simulink model "test_control_lib_poly_ctr_w_aw"  (R2017a)
settings: Solver=VariableStepAuto  StartTime=0.0  StopTime=0.020*100  RelTol=1e-3
libraries: simulink x11
settings Model: Creator=CHIVFUR  LastModifiedBy=CHIVFUR

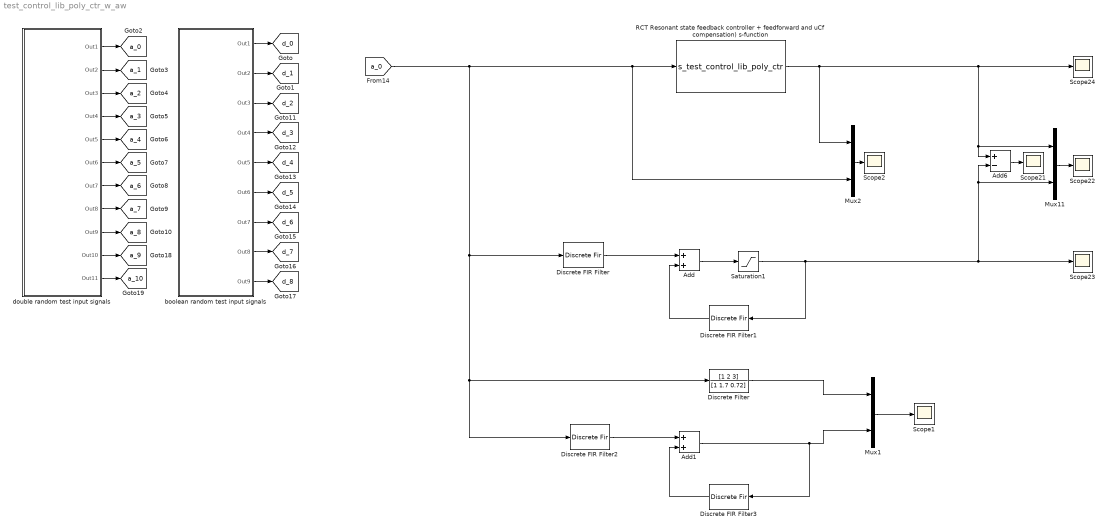
== system test_control_lib_poly_ctr_w_aw ==
  Add : Sum
  Add1 : Sum
  Add6 : Sum  Inputs=+-
  Discrete FIR Filter : DiscreteFir  Coefficients=[1 2 3]  SampleTime=1/30000
  Discrete FIR Filter1 : DiscreteFir  Coefficients=[0 -1.7 -0.72]  SampleTime=1/30000
  Discrete FIR Filter2 : DiscreteFir  Coefficients=[1 2 3]  SampleTime=1/30000
  Discrete FIR Filter3 : DiscreteFir  Coefficients=[0 -1.7 -0.72]  SampleTime=1/30000
  Discrete Filter : DiscreteFilter  Numerator=[1 2 3]  Denominator=[1 1.7 0.72]  SampleTime=1/30000
  Mux1 : Mux  Inputs=2
  Mux11 : Mux  Inputs=2
  Mux2 : Mux  Inputs=2
  RCT Resonant state feedback controller + feedforward and uCf compensation) s-function : S-Function  FunctionName=s_test_control_lib_poly_ctr  Parameters=1/30000,1.0  SFunctionDeploymentMode=off  EnableBusSupport=off
  Saturation1 : Saturate  UpperLimit=100  LowerLimit=-100
  Scope{1..2,21..24} (6 alike) : Scope
  boolean random test input signals : Subsystem
  double random test input signals : Subsystem
  tag scope: a_0=global, a_10=global, a_1=global, a_2=global, a_3=global, a_4=global, a_5=global, a_6=global, a_7=global, a_8=global, a_9=global, d_0=global, d_1=global, d_2=global, d_3=global, d_4=global, d_5=global, d_6=global, d_7=global, d_8=global
  wires:
  boolean random test input signals/2(Out2) -> [d_1]
  boolean random test input signals/1(Out1) -> [d_0]
  double random test input signals/1(Out1) -> [a_0]
  double random test input signals/2(Out2) -> [a_1]
  double random test input signals/3(Out3) -> [a_2]
  double random test input signals/4(Out4) -> [a_3]
  [a_0] -> Discrete FIR Filter/1, Discrete Filter/1, Discrete FIR Filter2/1, Mux2/2, RCT Resonant state feedback controller + feedforward and uCf compensation) s-function/1
  Add/1 -> Saturation1/1
  Add6/1 -> Scope21/1
  Mux11/1 -> Scope22/1
  double random test input signals/5(Out5) -> [a_4]
  double random test input signals/6(Out6) -> [a_5]
  double random test input signals/7(Out7) -> [a_6]
  double random test input signals/8(Out8) -> [a_7]
  double random test input signals/9(Out9) -> [a_8]
  boolean random test input signals/3(Out3) -> [d_2]
  boolean random test input signals/4(Out4) -> [d_3]
  boolean random test input signals/5(Out5) -> [d_4]
  boolean random test input signals/6(Out6) -> [d_5]
  boolean random test input signals/7(Out7) -> [d_6]
  boolean random test input signals/8(Out8) -> [d_7]
  boolean random test input signals/9(Out9) -> [d_8]
  double random test input signals/10(Out10) -> [a_9]
  double random test input signals/11(Out11) -> [a_10]
  Discrete FIR Filter1/1 -> Add/2
  RCT Resonant state feedback controller + feedforward and uCf compensation) s-function/1 -> Mux2/1, Scope24/1, Mux11/1, Add6/1
  Discrete FIR Filter/1 -> Add/1
  Discrete FIR Filter2/1 -> Add1/1
  Discrete FIR Filter3/1 -> Add1/2
  Discrete Filter/1 -> Mux1/1
  Add1/1 -> Discrete FIR Filter3/1, Mux1/2
  Mux1/1 -> Scope1/1
  Saturation1/1 -> Mux11/2, Add6/2, Scope23/1, Discrete FIR Filter1/1
  Mux2/1 -> Scope2/1

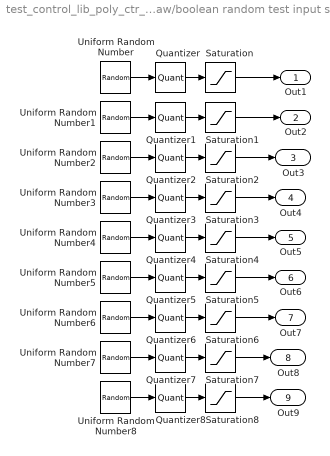
== system test_control_lib_poly_ctr_w_aw/boolean random test input signals ==
  Quantizer{,1..8} (9 alike) : Quantizer  QuantizationInterval=1
  Saturation{,1..8} (9 alike) : Saturate  UpperLimit=1  LowerLimit=0
  Uniform Random Number : UniformRandomNumber  Minimum=-4.5  Maximum=5.5  Seed=1  SampleTime=0.01
  Uniform Random Number1 : UniformRandomNumber  Minimum=-4.5  Maximum=5.5  Seed=2  SampleTime=0.01
  Uniform Random Number2 : UniformRandomNumber  Minimum=-4.5  Maximum=5.5  Seed=3  SampleTime=0.01
  Uniform Random Number3 : UniformRandomNumber  Minimum=-4.5  Maximum=5.5  Seed=4  SampleTime=0.01
  Uniform Random Number4 : UniformRandomNumber  Minimum=-4.5  Maximum=5.5  Seed=5  SampleTime=0.01
  Uniform Random Number5 : UniformRandomNumber  Minimum=-4.5  Maximum=5.5  Seed=6  SampleTime=0.01
  Uniform Random Number6 : UniformRandomNumber  Minimum=-4.5  Maximum=5.5  Seed=7  SampleTime=0.01
  Uniform Random Number7 : UniformRandomNumber  Minimum=-4.5  Maximum=5.5  Seed=8  SampleTime=0.01
  Uniform Random Number8 : UniformRandomNumber  Minimum=-4.5  Maximum=5.5  Seed=9  SampleTime=0.01
  Out1 : Outport
  Out2 : Outport  Port=2
  Out3 : Outport  Port=3
  Out4 : Outport  Port=4
  Out5 : Outport  Port=5
  Out6 : Outport  Port=6
  Out7 : Outport  Port=7
  Out8 : Outport  Port=8
  Out9 : Outport  Port=9
  wires:
  Uniform Random Number7/1 -> Quantizer7/1
  Quantizer7/1 -> Saturation7/1
  Quantizer6/1 -> Saturation6/1
  Uniform Random Number6/1 -> Quantizer6/1
  Uniform Random Number5/1 -> Quantizer5/1
  Quantizer5/1 -> Saturation5/1
  Quantizer4/1 -> Saturation4/1
  Uniform Random Number4/1 -> Quantizer4/1
  Uniform Random Number3/1 -> Quantizer3/1
  Quantizer3/1 -> Saturation3/1
  Quantizer2/1 -> Saturation2/1
  Uniform Random Number2/1 -> Quantizer2/1
  Uniform Random Number1/1 -> Quantizer1/1
  Quantizer1/1 -> Saturation1/1
  Quantizer/1 -> Saturation/1
  Uniform Random Number/1 -> Quantizer/1
  Saturation7/1 -> Out8/1
  Saturation6/1 -> Out7/1
  Saturation5/1 -> Out6/1
  Saturation4/1 -> Out5/1
  Saturation3/1 -> Out4/1
  Saturation2/1 -> Out3/1
  Saturation1/1 -> Out2/1
  Saturation/1 -> Out1/1
  Uniform Random Number8/1 -> Quantizer8/1
  Quantizer8/1 -> Saturation8/1
  Saturation8/1 -> Out9/1

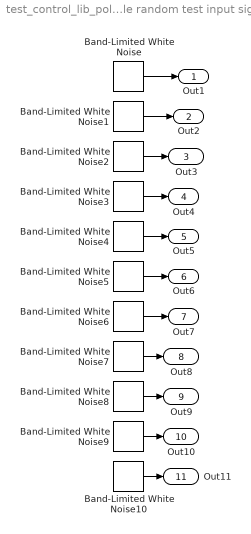
== system test_control_lib_poly_ctr_w_aw/double random test input signals ==
  Band-Limited White Noise : simulink/Sources/Band-Limited White Noise  Cov=[0.1]  Ts=1/30000  seed=1
  Band-Limited White Noise1 : simulink/Sources/Band-Limited White Noise  Cov=[0.1]  Ts=1/30000  seed=2
  Band-Limited White Noise10 : simulink/Sources/Band-Limited White Noise  Cov=[0.1]  Ts=1/30000  seed=11
  Band-Limited White Noise2 : simulink/Sources/Band-Limited White Noise  Cov=[0.1]  Ts=1/30000  seed=3
  Band-Limited White Noise3 : simulink/Sources/Band-Limited White Noise  Cov=[0.1]  Ts=1/30000  seed=4
  Band-Limited White Noise4 : simulink/Sources/Band-Limited White Noise  Cov=[0.1]  Ts=1/30000  seed=5
  Band-Limited White Noise5 : simulink/Sources/Band-Limited White Noise  Cov=[0.1]  Ts=1/30000  seed=6
  Band-Limited White Noise6 : simulink/Sources/Band-Limited White Noise  Cov=[0.1]  Ts=1/30000  seed=7
  Band-Limited White Noise7 : simulink/Sources/Band-Limited White Noise  Cov=[0.1]  Ts=1/30000  seed=8
  Band-Limited White Noise8 : simulink/Sources/Band-Limited White Noise  Cov=[0.1]  Ts=1/30000  seed=9
  Band-Limited White Noise9 : simulink/Sources/Band-Limited White Noise  Cov=[0.1]  Ts=1/30000  seed=10
  Out1 : Outport
  Out2 : Outport  Port=2
  Out3 : Outport  Port=3
  Out4 : Outport  Port=4
  Out5 : Outport  Port=5
  Out6 : Outport  Port=6
  Out7 : Outport  Port=7
  Out8 : Outport  Port=8
  Out9 : Outport  Port=9
  Out10 : Outport  Port=10
  Out11 : Outport  Port=11
  wires:
  Band-Limited White Noise4/1 -> Out5/1
  Band-Limited White Noise2/1 -> Out3/1
  Band-Limited White Noise/1 -> Out1/1
  Band-Limited White Noise5/1 -> Out6/1
  Band-Limited White Noise1/1 -> Out2/1
  Band-Limited White Noise6/1 -> Out7/1
  Band-Limited White Noise7/1 -> Out8/1
  Band-Limited White Noise3/1 -> Out4/1
  Band-Limited White Noise8/1 -> Out9/1
  Band-Limited White Noise9/1 -> Out10/1
  Band-Limited White Noise10/1 -> Out11/1
